simulink model "Computer_roe"  (R2018b)
settings: configuration reference "Configuration" (kept outside this file)
model workspace (MATLAB code in the model file):
  | CON = Simulink.Parameter;
  | CON.DataType = 'Bus: Bus_CON';
  | CON.Value = Simulink.Bus.createMATLABStruct('Bus_CON');
undefined symbols (not defined in the file): computer_dt
settings Model: ParameterArgumentNames=CON  OrderedModelArguments=off  Creator=Ethan  LastModifiedBy=Ethan
settings ConfigSetRef: SourceLocation=Base Workspace

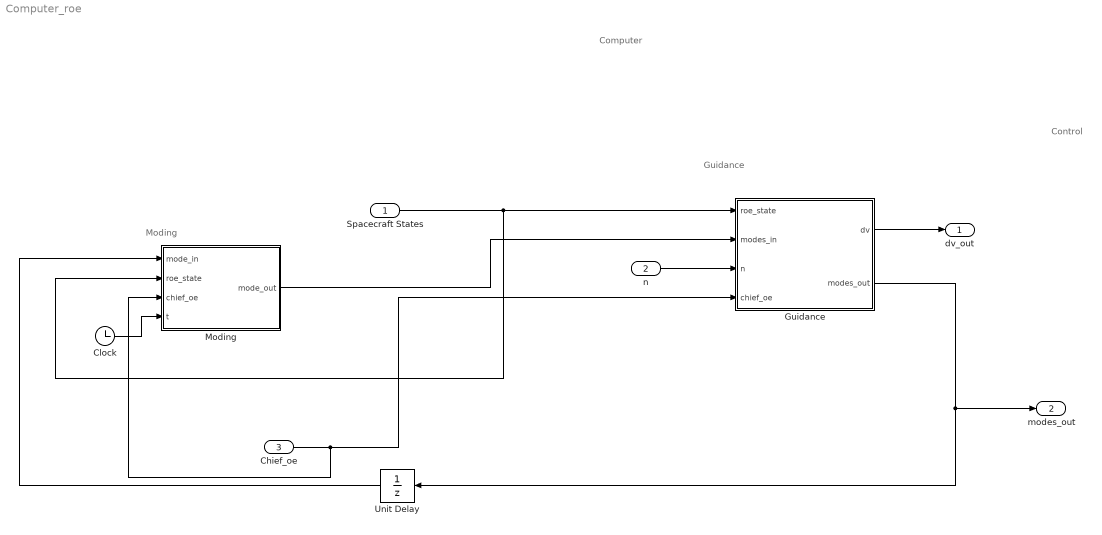
== system Computer_roe ==
  note: Computer
  note: Moding
  note: Control
  note: Guidance
  Spacecraft States : Inport  PortDimensions=7
  n : Inport  Port=2  PortDimensions=1
  Chief_oe : Inport  Port=3  OutDataTypeStr=Bus: Bus_OE  PortDimensions=1
  Clock : Clock
  Guidance : MATLAB Function  TreatAsAtomicUnit=on  SystemSampleTime=computer_dt
  Moding : MATLAB Function  TreatAsAtomicUnit=on  SystemSampleTime=computer_dt
  Unit Delay : UnitDelay  SampleTime=-1
  dv_out : Outport  PortDimensions=4
  modes_out : Outport  Port=2  OutDataTypeStr=Bus: Bus_modes
  wires:
  Spacecraft States/1 -> Moding/2(roe_state), Guidance/1(roe_state)
  Guidance/1(dv) -> dv_out/1
  Clock/1 -> Moding/4(t)
  Moding/1(mode_out) -> Guidance/2(modes_in)
  Guidance/2(modes_out) -> modes_out/1, Unit Delay/1
  Unit Delay/1 -> Moding/1(mode_in)
  n/1 -> Guidance/3(n)
  Chief_oe/1 -> Moding/3(chief_oe), Guidance/4(chief_oe)

== matlab function Computer_roe/Guidance ==
  data: roe_state input; modes_in input Bus: Bus_modes; n input; dv output; modes_out output Bus: Bus_modes; chief_oe input
function [dv, modes_out] = guid_bound_motion(roe_state, modes_in, n, chief_oe)
modes_out = modes_in;
dv = zeros(4, 1);


persistent dv_old
if isempty(dv_old)
    dv_old = zeros(4, 1);
end
desired_pos = [1, -15, 0]';

if modes_in.guid == 1
    [~, ud] = roe2Hill(roe_state, chief_oe);
    v_desired = -n * roe_state(2) * chief_oe.a / 2;
    dv = [0;v_desired;0; ud * pi / 180];
    modes_in.guid = 2;
    
% elseif modes_out.guid == 3
%     w = 80 * pi / 180;
%     t = w / n;
%     dv = cw_1burn(n, t, roe_state, desired_pos);
%     modes_in.guid = 4;
% elseif modes_out.guid == 5
%     dv = circ_burn(roe_state, n);
end
modes_out = modes_in;
dv_old = dv;
% dv = zeros(4, 1);
end

== matlab function Computer_roe/Moding ==
  data: mode_in input Bus: Bus_modes; roe_state input; chief_oe input; mode_out output Bus: Bus_modes; t input
function mode_out = moding(mode_in, roe_state, chief_oe, t)

mode_out  = mode_in; 
persistent tig_time
if isempty(tig_time)
    tig_time = 0;
end
desired_pos = [1, 0, 0]';
if any(roe_state ~= zeros(7, 1))
    rv_Hill = roe2Hill(roe_state, chief_oe);
    if rv_Hill(2) < -3 && mode_in.guid == 0
        mode_out.guid = 1;
    end
end
    
end
